simulink model "lookupnddirect_multi_complex_test"  (Simulink 8.4)
settings: Solver=ode45  StartTime=0.0  StopTime=10.0  RelTol=1e-3
settings Model: Creator=arnaud  LastModifiedBy=arnaud
settings DataIOCC: SaveFormat=Structure

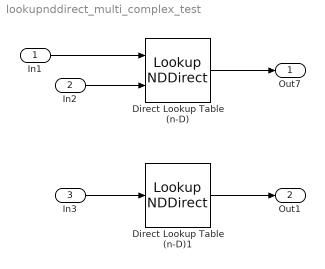
== system lookupnddirect_multi_complex_test ==
  In1 : Inport  PortDimensions=2
  In2 : Inport  Port=2  PortDimensions=2
  In3 : Inport  Port=3  PortDimensions=2
  Direct Lookup Table (n-D) : LookupNDDirect  Table=[4+5i 5+6i 6+7i;16+17i 19+20i 20+21i;10+11i 18+19i 23+24i]
  Direct Lookup Table (n-D)1 : LookupNDDirect  NumberOfTableDimensions=1  Table=[4+5i 5+6i 6+7i]
  Out7 : Outport
  Out1 : Outport  Port=2
  wires:
  In1/1 -> Direct Lookup Table (n-D)/1
  In2/1 -> Direct Lookup Table (n-D)/2
  Direct Lookup Table (n-D)/1 -> Out7/1
  In3/1 -> Direct Lookup Table (n-D)1/1
  Direct Lookup Table (n-D)1/1 -> Out1/1
